simulink model "sgMdl_ThermocoupleEmulation"  (R2024b)
settings: Solver=FixedStepAuto  StartTime=0.0  StopTime=inf  RelTol=1e-3  EnableMultiTasking=on
undefined symbols (not defined in the file): IO975, TypeJ_degC, TypeJ_Volts, TypeK_degC, TypeK_Volts
libraries: simulink x1, speedgoatlib_PIL x1
Description:
  | Thermocouple Emulation
settings Model: ModifiedByFormat=Speedgoat  SimulationMode=external  ExtModeTrigDuration=100000  Creator=Speedgoat  LastModifiedBy=Speedgoat
settings SolverCC: ConcurrentTasks=on  AlgebraicLoopSolver=TrustRegion  PositivePriorityOrder=on  InsertRTBMode=Never (minimum delay)
settings DataIOCC: SaveFormat=Array  SaveState=on  SignalLoggingName=logsOut
settings OptimizationCC: BlockReduction=off  BooleanDataType=off  OptimizeBlockIOStorage=off  BufferReuse=off  ReuseModelBlockBuffer=off  GlobalBufferReuse=off  ExpressionFolding=off  LocalBlockOutputs=off  InitFltsAndDblsToZero=on  OptimizeDataStoreBuffers=off  BusAssignmentInplaceUpdate=off
settings DebuggingCC: SaveWithParameterizedLinksMsg=none  UnderspecifiedInitializationDetection=Classic  MergeDetectMultiDrivingBlocksExec=none  CheckExecutionContextPreStartOutputMsg=on  SignalResolutionControl=TryResolveAllWithWarning  TasksWithSamePriorityMsg=none  UnconnectedInputMsg=warning  UnconnectedOutputMsg=warning  UnconnectedLineMsg=warning  SFUnexpectedBacktrackingDiag=warning  SFNoUnconditionalDefaultTransitionDiag=warning  SFExecutionAtInitializationDiag=none  ArithmeticOperatorsInVariantConditions=warning
settings HardwareCC: ProdBitPerLong=64  ProdLongLongMode=on  ProdHWDeviceType=Intel->x86-64 (Linux 64)
settings ModelReferenceCC: EnableRefExpFcnMdlSchedulingChecks=on  PropagateSignalLabelsOutOfModel=off
settings SFSimCC: SimUseLocalCustomCode=off  SimTargetLang=C++
settings RTWCC: Description=Speedgoat Real-Time Target Machine  SystemTargetFile=speedgoat.tlc  TemplateMakefile=slrealtime_default_tmf  PostCodeGenCommand=sg.model.build.makeCfg(bdroot, buildInfo);  RTWUseLocalCustomCode=off  Toolchain=Simulink Real-Time Toolchain  BuildConfiguration=Faster Runs  TargetLang=C++  GPUComputeCapability=3.5  DLArmComputeVersion=19.05
settings CodeAppCC: StateflowObjectComments=on
settings SimulinkRealTimeTargetCC: SubcomponentCodeInterfacePackaging=Reusable function  MATLABClassNameForMDSCustomization=Simulink.SoftwareTarget.GRTCustomization  InstructionSetFMA=off  LogToMDFFile=off  SLRTFileLogMaxRuns=10  UseGCCFastMath=on
settings ConfigComp: CovMetricSettings=dw  CovSaveCumulativeToWorkspaceVar=on  CovSaveSingleToWorkspaceVar=on  CovExternalEMLEnable=off  CovSFcnEnable=off  CovBoundaryAbsTol=1.0e-5

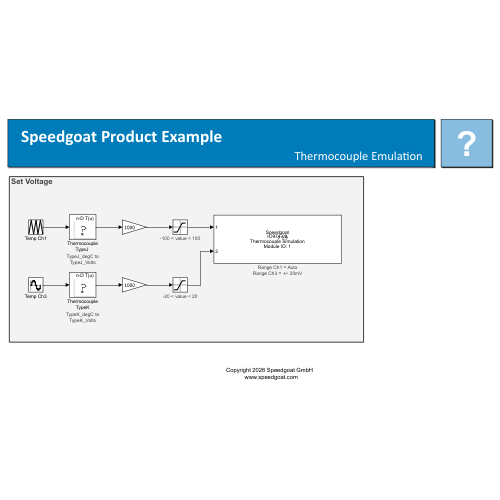
[thumbnail: Simulink's stored preview of the top-level diagram]
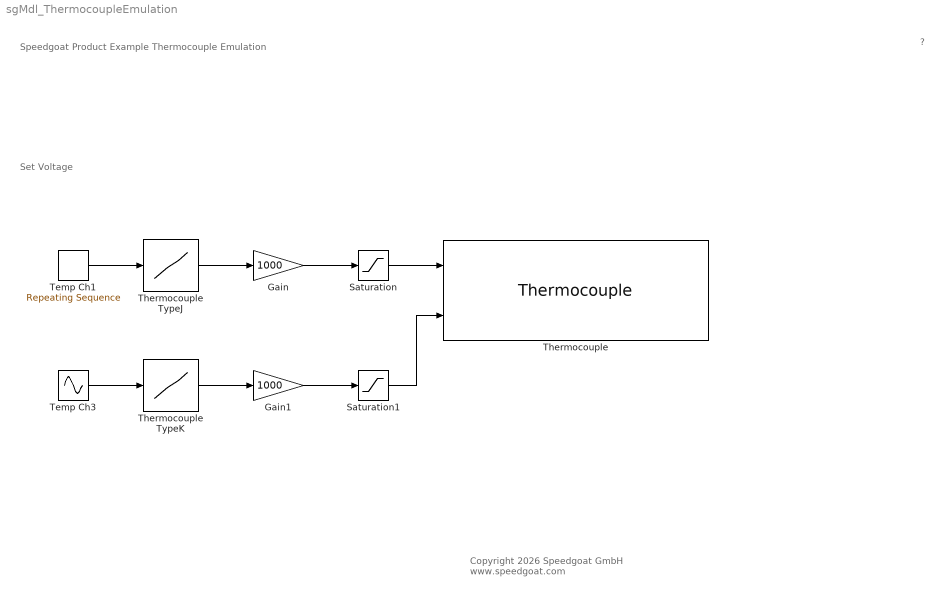
== system sgMdl_ThermocoupleEmulation ==
  note: Set Voltage
  note: Speedgoat Product Example
      | Thermocouple Emulation
  note: ?
  note: Copyright 2026 Speedgoat GmbH
      |  www.speedgoat.com
  Gain : Gain  Gain=1000
  Gain1 : Gain  Gain=1000
  Saturation : Saturate  UpperLimit=100  LowerLimit=-100
      settings: AttributesFormatString=%<LowerLimit> < value < %<UpperLimit>
  Saturation1 : Saturate  UpperLimit=20  LowerLimit=-20
      settings: AttributesFormatString=%<LowerLimit> < value < %<UpperLimit>
  Temp Ch1 : simulink/Sources/Repeating Sequence  rep_seq_t=[0 1 2]  rep_seq_y=[0 1200 0]
  Temp Ch3 : Sin  Amplitude=400  Frequency=0.5*pi  SampleTime=100e-3
  Thermocouple : speedgoatlib_PIL/Thermocouple  id=1  card_type=IO975-16  channel_vector=[1 3]  init_vector=[0 0]  reset_vector=[1 1]  range1=Auto  range2=+/- 20mV  range3=Auto  range4=Auto  range5=Auto  range6=Auto  range7=Auto  range8=Auto  enable_cold=on  enable_remote=on  ts=-1  slot=-1  range_vector=[0 0 1 1 0 0 0 0 0 0 0 0 0 0 0 0]  enChVec=[1 0 1 0 0 0 0 0 0 0 0 0 0 0 0 0]  enColdVec=[1 0 1 0 0 0 0 0 0 0 0 0 0 0 0 0]  enRemoteVec=[1 0 1 0 0 0 0 0 0 0 0 0 0 0 0 0]
      settings: SourceProductName=Simulink Real-Time: Speedgoat I/O Blockset
      settings: AttributesFormatString=|
      | Range Ch1 = %<range1>
      | Range Ch3 = %<range2>
  "Thermocouple TypeJ " : Lookup_n-D  NumberOfTableDimensions=1  BreakpointsForDimension1=TypeJ_degC  BeginIndexSearchUsingPreviousIndexResult=on  Table=TypeJ_Volts  DiagnosticForOutOfRangeInput=Warning
      settings: AttributesFormatString=%<bp1> to\n%<tableData>
  Thermocouple TypeK : Lookup_n-D  NumberOfTableDimensions=1  BreakpointsForDimension1=TypeK_degC  BeginIndexSearchUsingPreviousIndexResult=on  Table=TypeK_Volts  DiagnosticForOutOfRangeInput=Warning
      settings: AttributesFormatString=%<bp1> to\n%<tableData>
  wires:
  Temp Ch3/1 -> Thermocouple TypeK/1
  Temp Ch1/1 -> "Thermocouple TypeJ "/1
  Thermocouple TypeK/1 -> Gain1/1
  Gain1/1 -> Saturation1/1
  "Thermocouple TypeJ "/1 -> Gain/1
  Gain/1 -> Saturation/1
  Saturation/1 -> Thermocouple/1
  Saturation1/1 -> Thermocouple/2
